simulink model "simulink_observateur_luenberger_masse_ressort"  (R2018a)
settings: Solver=VariableStepAuto  StartTime=0.0  StopTime=20  RelTol=1e-3
InitFcn:
  | parametre
values from neighbouring files (symbols this model uses):
  A = [ 0      1 ... (first row only)    [parametre.m]
  B = [0;1/m]    [parametre.m]
  C = [1 0]    [parametre.m]
  L = Lt'    [parametre.m]
settings Model: Creator=Henin'T'soa  LastModifiedBy=Henin'T'soa

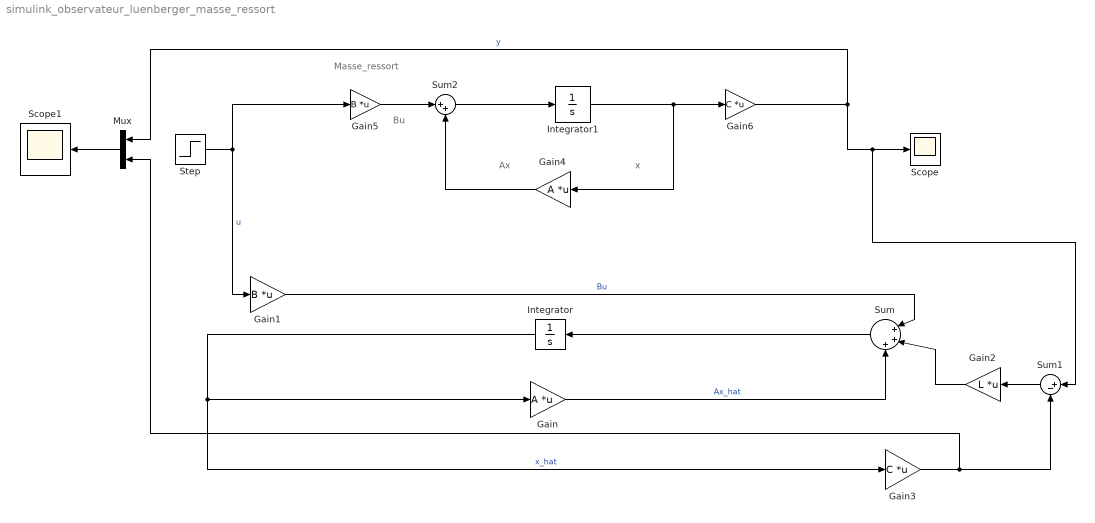
== system simulink_observateur_luenberger_masse_ressort ==
  note: Masse_ressort
  note: Ax
  note: x
  note: Bu
  Gain : Gain  Gain=A  Multiplication=Matrix(K*u)
  Gain1 : Gain  Gain=B  Multiplication=Matrix(K*u)
  Gain2 : Gain  Gain=L  Multiplication=Matrix(K*u)
  Gain3 : Gain  Gain=C  Multiplication=Matrix(K*u)
  Gain4 : Gain  Gain=A  Multiplication=Matrix(K*u)
  Gain5 : Gain  Gain=B  Multiplication=Matrix(K*u)
  Gain6 : Gain  Gain=C  Multiplication=Matrix(K*u)
  Integrator : Integrator  InitialCondition=[0.5;1]
  Integrator1 : Integrator  InitialCondition=[0;0.5]
  Mux : Mux  Inputs=2
  Scope : Scope
  Scope1 : Scope
  Step : Step  Time=0  SampleTime=0
  Sum : Sum  Inputs=|+++
  Sum1 : Sum  Inputs=|+-
  Sum2 : Sum  Inputs=|++
  wires:
  Step/1 -> Gain5/1, Gain1/1  "u"
  Integrator/1 -> Gain/1, Gain3/1  "x_hat"
  Gain/1 -> Sum/3  "Ax_hat"
  Gain1/1 -> Sum/1  "Bu"
  Gain2/1 -> Sum/2
  Sum1/1 -> Gain2/1
  Gain3/1 -> Mux/2, Sum1/2
  Sum/1 -> Integrator/1
  Mux/1 -> Scope1/1
  Gain4/1 -> Sum2/2
  Sum2/1 -> Integrator1/1
  Gain6/1 -> Sum1/1, Scope/1, Mux/1  "y"
  Integrator1/1 -> Gain6/1, Gain4/1
  Gain5/1 -> Sum2/1
